simulink model "MLS4_4_function_and_input_ycalcR2022b"  (R2022b)
settings: Solver=FixedStepAuto  StartTime=0.0  StopTime=5  FixedStep=0.01  RelTol=1e-3
undefined symbols (not defined in the file or in its folder): beta, calMp, lM, m4g, st0, xi
settings Model: Creator=Nico  LastModifiedBy=27658
settings OptimizationCC: ReuseModelBlockBuffer=on
settings DebuggingCC: UnderSpecifiedDimensionMsg=error
settings RTWCC: GPUComputeCapability=5.0

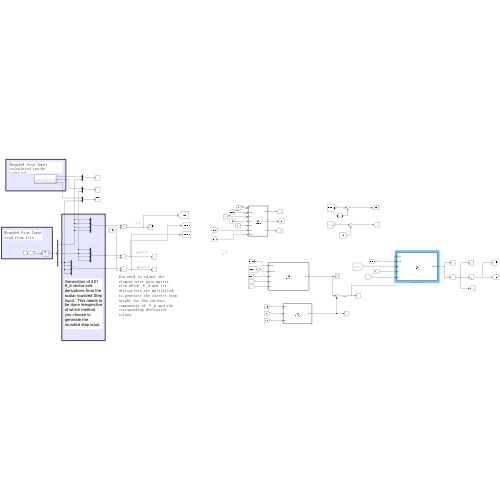
[thumbnail: Simulink's stored preview of the top-level diagram]
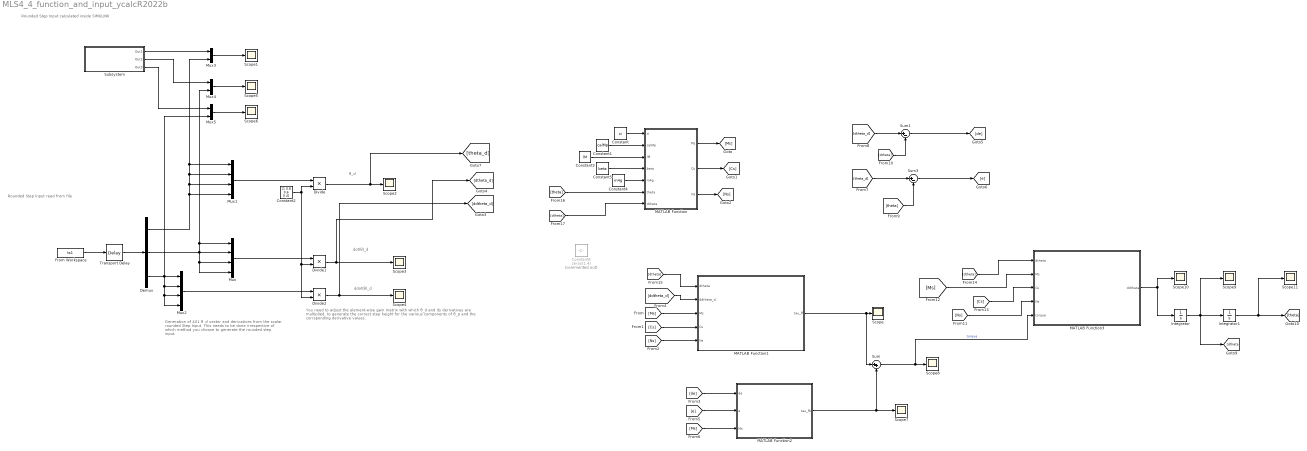
== system MLS4_4_function_and_input_ycalcR2022b ==
  note: You need to adjust the element-wise gain matrix with which θ_d and its derivatives are multiplied, to generate the correct step height for the various components of θ_p and the corrsponding derivative values.
  note: Generation of 4X1 θ_d vector and derivatives from the scalar rounded Step Input. This needs to be done irrespective of which method you choose to generate the rounded step input.
  note: Rounded Step Input
      | read from file
  note: Rounded Step Input
      | calculated inside SIMULINK
  note: ddot(θ)_d
  note: θ_d
  note: dot(θ)_d
  Constant : Constant  Value=xi
  Constant1 : Constant  Value=calMp
  Constant2 : Constant  Value=[1 0.8 0.6 0.4]
  Constant3 : Constant  Value=lM
  Constant4 : Constant  Value=m4g
  Constant5 : Constant  Value=beta
  Constant6 : Constant  Commented=on  Value=zeros(1,4)
  Demux : Demux  Outputs=3
  Divide : Product  Inputs=**
  Divide1 : Product  Inputs=**
  Divide2 : Product  Inputs=**
  From Workspace : FromWorkspace  VariableName=ts1
  Integrator : Integrator
  Integrator1 : Integrator
  MATLAB Function : MATLAB Function  TreatAsAtomicUnit=on
  MATLAB Function1 : MATLAB Function  TreatAsAtomicUnit=on
  MATLAB Function2 : MATLAB Function  TreatAsAtomicUnit=on
  MATLAB Function3 : MATLAB Function  TreatAsAtomicUnit=on
  Mux : Mux
  Mux1 : Mux
  Mux2 : Mux
  Mux3 : Mux  Inputs=2
  Mux4 : Mux  Inputs=2
  Mux5 : Mux  Inputs=2
  Scope{,1..11} (12 alike) : Scope
  Subsystem : Subsystem
  Sum : Sum  Inputs=|++
  Sum1 : Sum  Inputs=|+-
  Sum3 : Sum  Inputs=|+-
  Transport Delay : TransportDelay  DelayTime=[st0 st0 st0]
  wires:
  Mux2/1 -> Divide2/1
  Demux/1 -> Mux1/3, Mux1/2, Mux3/2, Mux1/1, Mux1/4
  Demux/2 -> Mux/4, Mux/3, Mux4/2, Mux/1, Mux/2
  Demux/3 -> Mux5/2, Mux2/2, Mux2/3, Mux2/4, Mux2/1
  Mux1/1 -> Divide/1
  Mux/1 -> Divide1/1
  Constant2/1 -> Divide2/2, Divide1/2, Divide/2
  Divide/1 -> [theta_d], Scope2/1
  Divide1/1 -> [dtheta_d], Scope3/1
  Divide2/1 -> [ddtheta_d], Scope4/1
  Constant/1 -> MATLAB Function/1(xi)
  Constant1/1 -> MATLAB Function/2(calMp)
  Constant3/1 -> MATLAB Function/3(lM)
  Constant4/1 -> MATLAB Function/5(m4g)
  Constant5/1 -> MATLAB Function/4(beta)
  Mux3/1 -> Scope1/1
  Subsystem/1(Out1) -> Mux3/1
  Subsystem/2(Out2) -> Mux4/1
  Subsystem/3(Out3) -> Mux5/1
  Mux4/1 -> Scope5/1
  Mux5/1 -> Scope6/1
  From Workspace/1 -> Transport Delay/1
  Transport Delay/1 -> Demux/1
  MATLAB Function1/1(tau_ff) -> Sum/1, Scope/1
  MATLAB Function/1(Ms) -> [Ms]
  MATLAB Function/2(Cs) -> [Cs]
  MATLAB Function/3(Ns) -> [Ns]
  [Ms] -> MATLAB Function1/3(Ms)
  [Cs] -> MATLAB Function1/4(Cs)
  [Ns] -> MATLAB Function1/5(Ns)
  [ddtheta_d] -> MATLAB Function1/2(ddtheta_d)
  MATLAB Function2/1(tau_fb) -> Sum/2, Scope7/1
  Sum/1 -> Scope8/1, MATLAB Function3/5(torque)  "torque"
  [de] -> MATLAB Function2/1(de)
  [e] -> MATLAB Function2/2(e)
  [Ms] -> MATLAB Function2/3(Ms)
  [theta_d] -> Sum3/1
  Sum3/1 -> [e]
  [dtheta_d] -> Sum1/1
  [dtheta] -> Sum1/2
  [theta] -> Sum3/2
  Sum1/1 -> [de]
  MATLAB Function3/1(ddtheta) -> Scope10/1, Integrator/1
  Integrator/1 -> Integrator1/1, [dtheta], Scope9/1
  Integrator1/1 -> [theta], Scope11/1
  [dtheta] -> MATLAB Function1/1(dtheta)
  [theta] -> MATLAB Function/6(theta)
  [dtheta] -> MATLAB Function/7(dtheta)
  [Ms] -> MATLAB Function3/2(Ms)
  [dtheta] -> MATLAB Function3/1(dtheta)
  [Ns] -> MATLAB Function3/4(Ns)
  [Cs] -> MATLAB Function3/3(Cs)

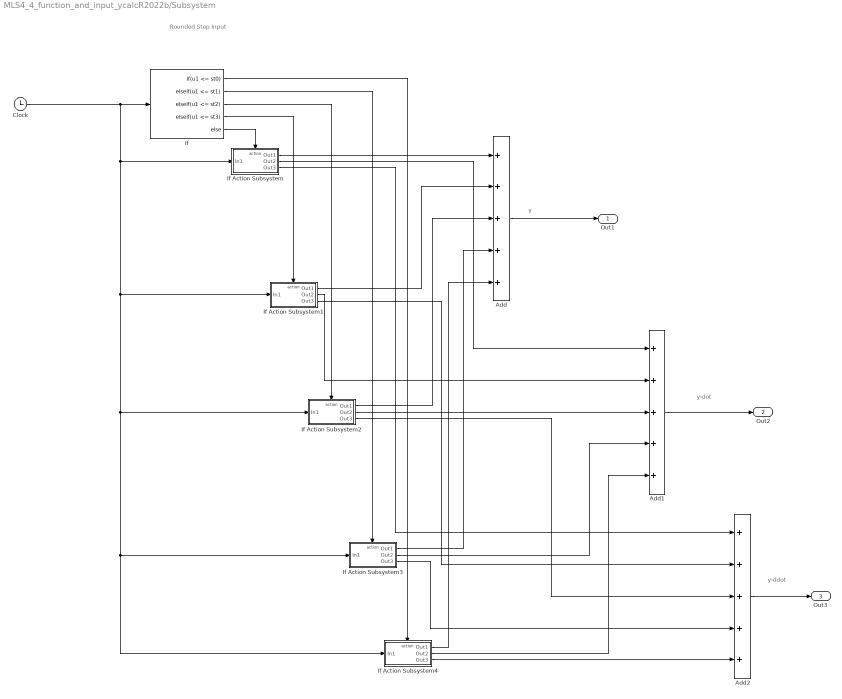
== system MLS4_4_function_and_input_ycalcR2022b/Subsystem ==
  note: Rounded Step Input
  note: y-ddot
  note: y-dot
  note: y
  Add : Sum  Inputs=+++++
  Add1 : Sum  Inputs=+++++
  Add2 : Sum  Inputs=+++++
  Clock : Clock
  If : If  IfExpression=u1 <= st0  ElseIfExpressions=u1 <= st1, u1 <= st2, u1 <= st3
  If Action Subsystem : Subsystem  TreatAsAtomicUnit=on
  If Action Subsystem1 : Subsystem  TreatAsAtomicUnit=on
  If Action Subsystem2 : Subsystem  TreatAsAtomicUnit=on
  If Action Subsystem3 : Subsystem  TreatAsAtomicUnit=on
  If Action Subsystem4 : Subsystem  TreatAsAtomicUnit=on
  Out1 : Outport
  Out2 : Outport  Port=2
  Out3 : Outport  Port=3
  wires:
  If Action Subsystem1/1(Out1) -> Add/2
  If/5 -> If Action Subsystem/Action
  If/3 -> If Action Subsystem2/Action
  If/2 -> If Action Subsystem3/Action
  If Action Subsystem/1(Out1) -> Add/1
  If Action Subsystem4/1(Out1) -> Add/5
  If/4 -> If Action Subsystem1/Action
  If/1 -> If Action Subsystem4/Action
  If Action Subsystem3/1(Out1) -> Add/4
  If Action Subsystem2/1(Out1) -> Add/3
  Add/1 -> Out1/1
  Add1/1 -> Out2/1
  Add2/1 -> Out3/1
  Clock/1 -> If Action Subsystem4/1(In1), If Action Subsystem3/1(In1), If Action Subsystem2/1(In1), If Action Subsystem1/1(In1), If Action Subsystem/1(In1), If/1
  If Action Subsystem/2(Out2) -> Add1/1
  If Action Subsystem/3(Out3) -> Add2/1
  If Action Subsystem1/2(Out2) -> Add1/2
  If Action Subsystem1/3(Out3) -> Add2/2
  If Action Subsystem2/2(Out2) -> Add1/3
  If Action Subsystem2/3(Out3) -> Add2/3
  If Action Subsystem3/3(Out3) -> Add2/4
  If Action Subsystem3/2(Out2) -> Add1/4
  If Action Subsystem4/2(Out2) -> Add1/5
  If Action Subsystem4/3(Out3) -> Add2/5

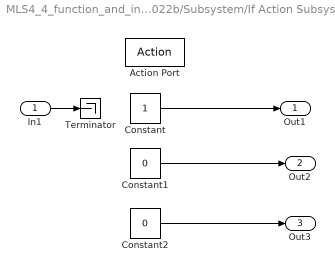
== system MLS4_4_function_and_input_ycalcR2022b/Subsystem/If Action Subsystem ==
  In1 : Inport
  Action Port : ActionPort  ActionPortLabel=else
  Constant : Constant
  Constant1 : Constant  Value=0
  Constant2 : Constant  Value=0
  Terminator : Terminator
  Out1 : Outport  OutputWhenDisabled=reset  InitialOutput=0
  Out2 : Outport  Port=2  OutputWhenDisabled=reset  InitialOutput=0
  Out3 : Outport  Port=3
  wires:
  Constant/1 -> Out1/1
  In1/1 -> Terminator/1
  Constant1/1 -> Out2/1
  Constant2/1 -> Out3/1

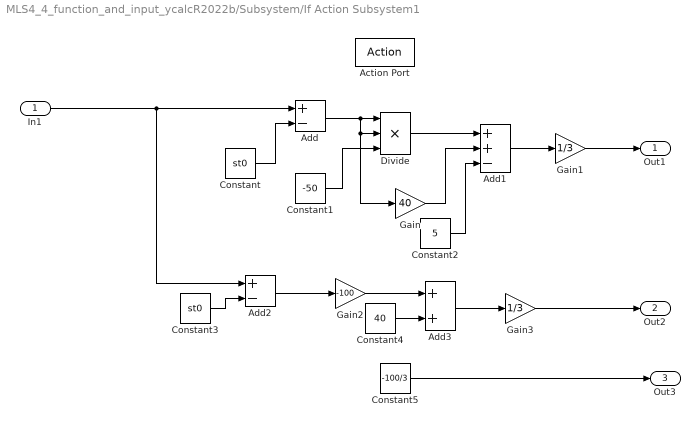
== system MLS4_4_function_and_input_ycalcR2022b/Subsystem/If Action Subsystem1 ==
  In1 : Inport
  Action Port : ActionPort  ActionPortLabel=elseif( u1 <= st3)
  Add : Sum  Inputs=+-
  Add1 : Sum  Inputs=++-
  Add2 : Sum  Inputs=+-
  Add3 : Sum
  Constant : Constant  Value=st0
  Constant1 : Constant  Value=-50
  Constant2 : Constant  Value=5
  Constant3 : Constant  Value=st0
  Constant4 : Constant  Value=40
  Constant5 : Constant  Value=-100/3
  Divide : Product  Inputs=***
  Gain : Gain  Gain=40
  Gain1 : Gain  Gain=1/3
  Gain2 : Gain  Gain=-100
  Gain3 : Gain  Gain=1/3
  Out1 : Outport  OutputWhenDisabled=reset  InitialOutput=0
  Out2 : Outport  Port=2  OutputWhenDisabled=reset  InitialOutput=0
  Out3 : Outport  Port=3  OutputWhenDisabled=reset  InitialOutput=0
  wires:
  In1/1 -> Add2/1, Add/1
  Constant1/1 -> Divide/3
  Constant/1 -> Add/2
  Add/1 -> Gain/1, Divide/2, Divide/1
  Divide/1 -> Add1/1
  Gain/1 -> Add1/2
  Constant2/1 -> Add1/3
  Add1/1 -> Gain1/1
  Gain1/1 -> Out1/1
  Add2/1 -> Gain2/1
  Gain2/1 -> Add3/1
  Add3/1 -> Gain3/1
  Constant3/1 -> Add2/2
  Constant4/1 -> Add3/2
  Gain3/1 -> Out2/1
  Constant5/1 -> Out3/1

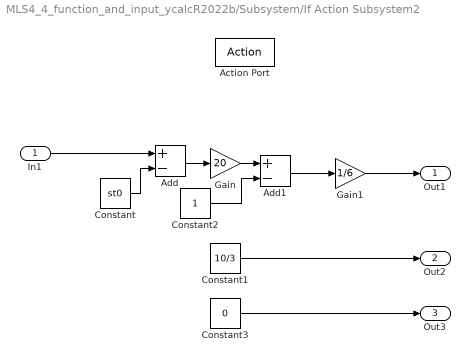
== system MLS4_4_function_and_input_ycalcR2022b/Subsystem/If Action Subsystem2 ==
  In1 : Inport
  Action Port : ActionPort  ActionPortLabel=elseif( u1 <= st2)
  Add : Sum  Inputs=+-
  Add1 : Sum  Inputs=+-
  Constant : Constant  Value=st0
  Constant1 : Constant  Value=10/3
  Constant2 : Constant
  Constant3 : Constant  Value=0
  Gain : Gain  Gain=20
  Gain1 : Gain  Gain=1/6
  Out1 : Outport  OutputWhenDisabled=reset  InitialOutput=0
  Out2 : Outport  Port=2  OutputWhenDisabled=reset  InitialOutput=0
  Out3 : Outport  Port=3  OutputWhenDisabled=reset  InitialOutput=0
  wires:
  In1/1 -> Add/1
  Constant/1 -> Add/2
  Add/1 -> Gain/1
  Gain/1 -> Add1/1
  Constant2/1 -> Add1/2
  Add1/1 -> Gain1/1
  Gain1/1 -> Out1/1
  Constant1/1 -> Out2/1
  Constant3/1 -> Out3/1

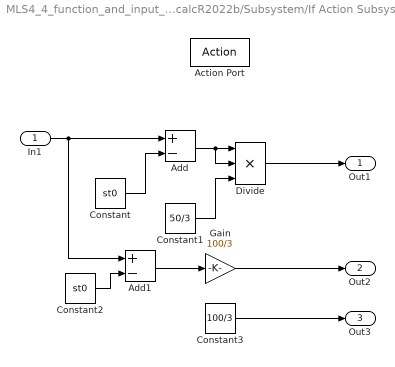
== system MLS4_4_function_and_input_ycalcR2022b/Subsystem/If Action Subsystem3 ==
  In1 : Inport
  Action Port : ActionPort  ActionPortLabel=elseif(u1 <= st1)
  Add : Sum  Inputs=+-
  Add1 : Sum  Inputs=+-
  Constant : Constant  Value=st0
  Constant1 : Constant  Value=50/3
  Constant2 : Constant  Value=st0
  Constant3 : Constant  Value=100/3
  Divide : Product  Inputs=***
  Gain : Gain  Gain=100/3
  Out1 : Outport  OutputWhenDisabled=reset  InitialOutput=0
  Out2 : Outport  Port=2  OutputWhenDisabled=reset  InitialOutput=0
  Out3 : Outport  Port=3  OutputWhenDisabled=reset  InitialOutput=0
  wires:
  In1/1 -> Add1/1, Add/1
  Constant/1 -> Add/2
  Add/1 -> Divide/2, Divide/1
  Constant1/1 -> Divide/3
  Divide/1 -> Out1/1
  Add1/1 -> Gain/1
  Constant2/1 -> Add1/2
  Gain/1 -> Out2/1
  Constant3/1 -> Out3/1

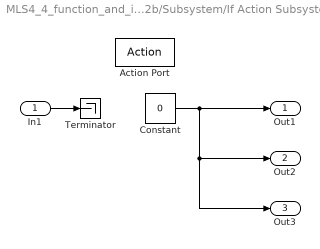
== system MLS4_4_function_and_input_ycalcR2022b/Subsystem/If Action Subsystem4 ==
  In1 : Inport
  Action Port : ActionPort  ActionPortLabel=if(u1 <= st0)
  Constant : Constant  Value=0
  Terminator : Terminator
  Out1 : Outport  OutputWhenDisabled=reset  InitialOutput=0
  Out2 : Outport  Port=2  OutputWhenDisabled=reset  InitialOutput=0
  Out3 : Outport  Port=3  OutputWhenDisabled=reset  InitialOutput=0
  wires:
  Constant/1 -> Out2/1, Out3/1, Out1/1
  In1/1 -> Terminator/1

== matlab function MLS4_4_function_and_input_ycalcR2022b/MATLAB Function1 ==
  data: dtheta input; tau_ff output; ddtheta_d input; Ms input; Cs input; Ns input
function tau_ff = Torque_ff(dtheta, ddtheta_d, Ms, Cs, Ns)

  tau_ff = Ms * ddtheta_d + Cs * dtheta + Ns;
end

== matlab function MLS4_4_function_and_input_ycalcR2022b/MATLAB Function ==
  data: xi input; Ms output; calMp input; lM input; beta input; m4g input; theta input; dtheta input; Cs output; Ns output
function [Ms,Cs,Ns] = MCNsim(xi,calMp,lM,beta,m4g,theta,dtheta)
    %%
    % We calculate $e^{\hat{\xi}\theta}$ for each joint.
    gg = zeros(4,4,4);
    gg(1:4,1:4,1) = gtwist_num(xi(:,1),theta(1));
    gg(1:4,1:4,2) = gtwist_num(xi(:,2),theta(2));
    gg(1:4,1:4,3) = gtwist_num(xi(:,3),theta(3));
    gg(1:4,1:4,4) = gtwist_num(xi(:,4),theta(4));
    %%  
    % Calculation of all possible $A_{lj}$ and all possible $A_{lj}\xi_j$
    Alj = zeros(6,6,4,4);
    Al  = zeros(6,4,4);
    for jj = 1:4
        for ll = 1:4
            ggjl = eye(4);
            for kk = jj+1:ll
                ggjl = ggjl*gg(:,:,kk);
            end
            dum        = adjmginv(ggjl);
            Alj(1:6,1:6,ll,jj) = dum;
            Al(1:6,ll,jj)  = dum*xi(:,jj);
        end
    end
    %% 
    % Calculation of $M(\theta)$ without utilizing the fact that it is
    %    symmetric.
    M = zeros(4);
    for ii = 1:4
        for jj = 1:4
            for ll = lM(ii,jj):4
                M(ii,jj) = M(ii,jj) + ...
                    Al(1:6,ll,ii)'*calMp(1:6,1:6,ll)*Al(1:6,ll,jj);
            end
        end
    end
    %% 
    % Calculation of
    % 
    % $$\frac{\partial M_{ij}}{\partial \theta_k}$$
    Ck  = zeros(4,4,4);
    for kk = 1:4
        Ckk = zeros(4,4);
        for ii = 1:4
            for jj = 1:4
                for ll = lM(ii,jj):4
                    dumii = Alkliejk_nca(Alj,Al,xi,ll,kk,ii);
                    dumjj = Alkliejk_nca(Alj,Al,xi,ll,kk,jj);
                    
                    Ckk(ii,jj) = Ckk(ii,jj) + ...
                    dumii'*calMp(1:6,1:6,ll)*Al(1:6,ll,jj) + ...
                    Al(1:6,ll,ii)'*calMp(1:6,1:6,ll)*dumjj;
                end
            end
        end
        Ck(1:4,1:4,kk) = Ckk;
    end
    %% 
    % Calculation of $C(\theta,\dot{\theta})$
    C = zeros(4);
    for ii = 1:4
        for jj = 1:4
            dum = 0;
            for kk = 1:4
                dum = dum + ( Ck(ii,jj,kk) + Ck(ii,kk,jj) - ...
                      Ck(kk,jj,ii) )*dtheta(kk);
            end
            C(ii,jj) = dum/2;
        end
    end
    %%
    % Caculation of $N(\theta,\dot{\theta})$
    N    = zeros(4,1);
    N(1) = beta(1)*dtheta(1);
    N(2) = beta(2)*dtheta(2);
    N(3) = beta(3)*dtheta(3);
    N(4) = beta(4)*dtheta(4) + m4g;

    Ms = M;
    Cs = C;
    Ns = N;
end

== matlab function MLS4_4_function_and_input_ycalcR2022b/MATLAB Function2 ==
  data: de input; tau_fb output; e input; Ms input
function tau_fb = Torque_fb(de, e, Ms)
zeta = 0.707;
Ts   = 1.2;             % desired settling time [s]
wn   = 4/(zeta*Ts);     % ≈4.7 rad/s

Kp = diag([wn^2, wn^2, wn^2, wn^2]);      
Kv = diag([2*zeta*wn, 2*zeta*wn, 2*zeta*wn, 2*zeta*wn]);  

Kv = [4.6 0 0 0;0 4.6 0 0;0 0 4.6 0;0 0 0 4.6]
Kp = [19.79660611840254 0 0 0;0 19.79660611840254 0 0;0 0 19.79660611840254 0;0 0 0 15.137455796741383]

tau_fb = Ms * (-Kv * de - Kp * e);
end

== matlab function MLS4_4_function_and_input_ycalcR2022b/MATLAB Function3 ==
  data: dtheta input; Ms input; Cs input; Ns input; torque input; ddtheta output
function ddtheta = ddtheta( dtheta, Ms, Cs, Ns, torque)

  ddtheta = Ms \ (torque - Cs * dtheta - Ns);
end
